simulink model "EvBoltCalib_Lat_v1_comb"  (R2022b)
settings: configuration reference "ConfigSetDesktopFixedStep" (kept outside this file)
PreLoadFcn:
  | VSS_BICYCLE=Simulink.Variant('Dual=0');
  | VSS_DUAL=Simulink.Variant('Dual=1');
  | Dual=1;
undefined symbols (not defined in the file or in its folder): BattChargeLimitMaxPwr, BattChargeLimitSocBpts, BattChargeLimitTbl, BattChrgCapcty, BattDischargeLimitSocBpts, BattDischargeLimitTbl, BattDischargeMaxPwr, BattNumCellsParallel, BattNumCellsSeries, BattOpenVoltCapBpts, BattOpenVoltTbl, BattResistSocBpts, BattResistTbl, BattResistTempBpts, BrakeMaxPrs, BrakeMaxTrq, ChassisDistCg2FrontAxle, ChassisDistCg2RearAxle, ChassisVehMass, DiffRatio, EnvGravCnst, EnvPrs, EnvTemp, ExpRefStructs, FuelSpecificGrav, h, InitStates, MtrEffSpdBpts, MtrEffTbl, MtrEffTrqBpts, MtrPwrMax, MtrTrqMax, SupvsryCtrlRegenBrkCutOffTbl, SupvsryCtrlRegenSpdBpts, TestScnrioCycleNum, VEH
libraries: vehdynlibtire x8, vehdynlibsuspension x7, autolibshared x6, simulink x6, autolibutils x5, VsrLibWheel x4, vehdynlibtirecommon x3, sharedtransform x3, autolibbatterycommon x2, autolibpowerinfoutils x2, autolibsharedcoupling x2, LibPtSupervisoryCtrl x2
(part 1 of 9)
settings Model: DataDictionary=DdPassengerEv.sldd  EnableAccessToBaseWorkspace=off  SimulationMode=accelerator  PauseTimes=45  Creator=9bt  LastModifiedBy=4qz
settings ConfigSetRef: SourceName=ConfigSetDesktopFixedStep

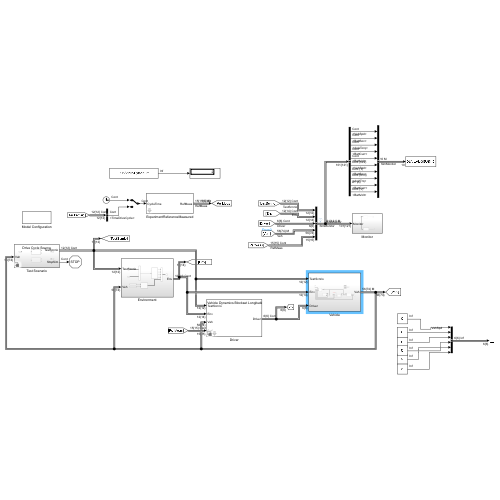
[thumbnail: Simulink's stored preview of the top-level diagram]
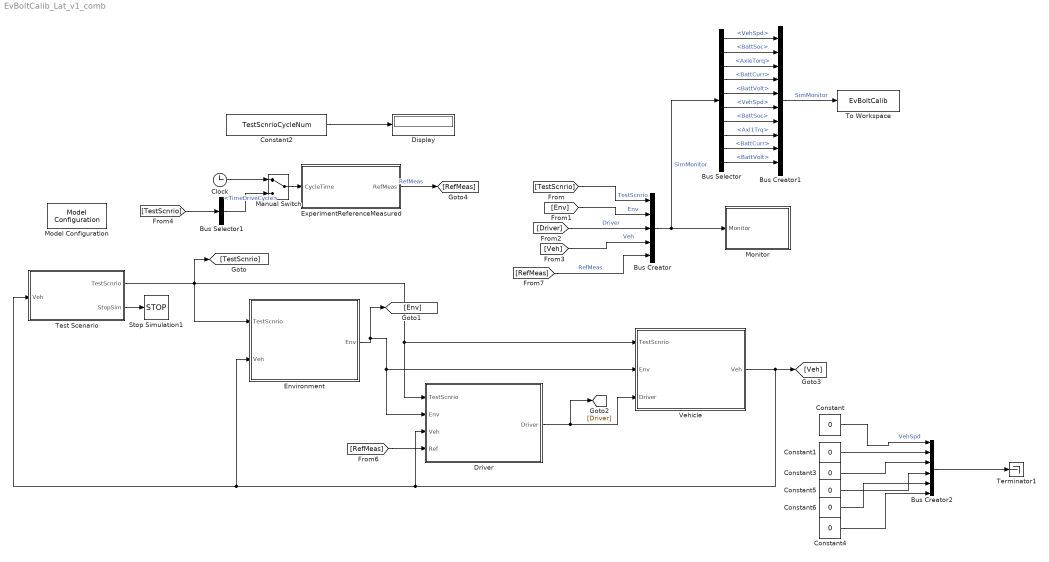
== system EvBoltCalib_Lat_v1_comb ==
  Bus Creator : BusCreator  Inputs=5
  Bus Creator1 : BusCreator  Inputs=10
  Bus Creator2 : BusCreator  Inputs=6
  Bus Selector : BusSelector  OutputSignals=RefMeas.VehSpd,RefMeas.BattSoc,RefMeas.AxleTorq,RefMeas.BattCurr,RefMeas.BattVolt,Veh.Chassis.VehSpd,Veh.Batt.BattSoc,Veh.Diff.Axl1.Axl1Trq,Veh.Batt.BattCurr,Veh.Batt.BattVolt
  Bus Selector1 : BusSelector  OutputSignals=TimeDriveCycle
  Clock : Clock
  Constant{,1,3..6} (6 alike) : Constant  Value=0
  Constant2 : Constant  Value=TestScnrioCycleNum
  Display : Display
  Driver : Subsystem  Variant=on  VariantControlMode=label  LabelModeActiveChoice=VdbLongDriver  mask{DriverSel=Vehicle Dynamics Blockset Longitudinal Driver}
      mask prompts: DriverSel "Select the driver"
      mask init:
      | choice = get_param(gcb,'DriverSel');
      | vssBlk = gcb;
      | oldVariant = get_param(gcb,'LabelModeActiveChoice');
      | switch choice
      |     case 'Predictive Longitudinal Driver'
      |         set_param(vssBlk, 'LabelModeActiveChoice', 'PredDriver');
      |     case 'Open Loop Driver'   
      |         set_param(vssBlk, 'LabelModeActiveChoice', 'OpenLoopDriver');
      |     case 'Direct Command From Reference'   
      |         set_param(vssBlk, 'LabelModeActiveChoice', 'DirectRef');
      |     case 'Vehicle Dynamics Blockset Longitudinal Driver'   
      |         set_param(vssBlk, 'LabelModeActiveChoice', 'VdbLongDriver');
      |     case 'Vehicle Dynamics Blockset Complete Driver'   
      |         set_param(vssBlk, 'LabelModeActiveChoice', 'VdbCompDriver');  
      | end
      mask TypeOptions DriverSel: Predictive Longitudinal Driver | Open Loop Driver | Direct Command From Reference | Vehicle Dynamics Blockset Longitudinal Driver | Vehicle Dynamics Blockset Complete Driver
  Environment : Subsystem
  ExperimentReferenceMeasured : Subsystem  mask{TestScnrioCycleNum=TestScnrioCycleNum, ExpRefStructs=ExpRefStructs}
      mask prompts: TestScnrioCycleNum "Driving Cycle Number"; ExpRefStructs "Experiment Reference Struct from Data Dictionary"
      mask init:
      | obj = ExpRefBlkCtrl(gcb);
      | MaskData = obj.Init;
      mask DialogControl Container3 Prompt: Parameters
  Manual Switch : ManualSwitch
  Model Configuration : VsrLibMdlConfig/Model Configuration  ConfigFileName=getMdlConfigs
  Monitor : Subsystem
  Stop Simulation1 : Stop
  Terminator1 : Terminator
  Test Scenario : Subsystem  Variant=on  VariantControlMode=label  LabelModeActiveChoice=DriveCycleSrc
  To Workspace : ToWorkspace  VariableName=EvBoltCalib  SaveFormat=Structure With Time  SampleTime=-1
  Vehicle : Subsystem
  wires:
  Driver/1(Driver) -> [Driver], Vehicle/3(Driver)
  Environment/1(Env) -> [Env], Driver/2(Env), Vehicle/2(Env)
  [TestScnrio] -> Bus Creator/1  "TestScnrio"
  [Env] -> Bus Creator/2  "Env"
  Test Scenario/2(StopSim) -> Stop Simulation1/1
  [RefMeas] -> Bus Creator/5  "RefMeas"
  Test Scenario/1(TestScnrio) -> [TestScnrio], Driver/1(TestScnrio), Vehicle/1(TestScnrio), Environment/1(TestScnrio)
  [RefMeas] -> Driver/4(Ref)
  ExperimentReferenceMeasured/1(RefMeas) -> [RefMeas]  "RefMeas"
  [TestScnrio] -> Bus Selector1/1
  Manual Switch/1 -> ExperimentReferenceMeasured/1(CycleTime)
  Clock/1 -> Manual Switch/1
  Bus Selector1/1 -> Manual Switch/2  "<TimeDriveCycle>"
  Constant2/1 -> Display/1
  Bus Selector/5 -> Bus Creator1/5  "<BattVolt>"
  Bus Creator1/1 -> To Workspace/1  "SimMonitor"
  Bus Selector/6 -> Bus Creator1/6  "<VehSpd>"
  Bus Selector/10 -> Bus Creator1/10  "<BattVolt>"
  Bus Selector/7 -> Bus Creator1/7  "<BattSoc>"
  Bus Selector/8 -> Bus Creator1/8  "<Axl1Trq>"
  Bus Selector/4 -> Bus Creator1/4  "<BattCurr>"
  Bus Selector/2 -> Bus Creator1/2  "<BattSoc>"
  Bus Selector/3 -> Bus Creator1/3  "<AxleTorq>"
  Bus Selector/1 -> Bus Creator1/1  "<VehSpd>"
  Bus Selector/9 -> Bus Creator1/9  "<BattCurr>"
  Bus Creator/1 -> Monitor/1(Monitor), Bus Selector/1  "SimMonitor"
  [Driver] -> Bus Creator/3  "Driver"
  [Veh] -> Bus Creator/4  "Veh"
  Constant/1 -> Bus Creator2/1  "VehSpd"
  Vehicle/1(Veh) -> Environment/2(Veh), Test Scenario/1(Veh), Driver/3(Veh), [Veh]
  Constant1/1 -> Bus Creator2/2
  Constant3/1 -> Bus Creator2/3
  Constant4/1 -> Bus Creator2/6
  Constant5/1 -> Bus Creator2/4
  Constant6/1 -> Bus Creator2/5
  Bus Creator2/1 -> Terminator1/1

== system EvBoltCalib_Lat_v1_comb/Driver ==
  TestScnrio : Inport
  Env : Inport  Port=2
  Veh : Inport  Port=3
  Ref : Inport  Port=4
  Direct Command From Reference : Subsystem  VariantControl=DirectRef
  Open Loop Driver : Subsystem  VariantControl=OpenLoopDriver
  Predictive Longitudinal Driver : Subsystem  VariantControl=PredDriver
  Vehicle Dynamics Blockset Complete Driver : Subsystem  VariantControl=VdbCompDriver
  "Vehicle Dynamics Blockset Longitudinal Driver " : Subsystem  VariantControl=VdbLongDriver
  Driver : Outport

== system EvBoltCalib_Lat_v1_comb/Environment ==
  TestScnrio : Inport
  Veh : Inport  Port=2
  Friction : Constant  Value=ones(4,1).*1
  Ground Feedback : Subsystem  Variant=on  VariantControlMode=label  LabelModeActiveChoice=0
  Ground Z Level : Constant  Value=zeros(4,1)
  Subsystem : Subsystem
  Subsystem1 : Subsystem
      mask Display: disp('')
  Subsystem2 : Subsystem
      mask Display: disp('')
  Env : Outport
  wires:
  Veh/1 -> Subsystem2/2(Veh)
  Subsystem/3(WindVel) -> Subsystem1/3(WindVel)
  Subsystem/2(EnvTemp) -> Subsystem1/2(EnvTemp)
  Subsystem/4(RoadGrade) -> Subsystem1/4(RoadGrade)
  Subsystem/1(EnvPrs) -> Subsystem1/1(EnvPrs)
  Subsystem1/1(Env) -> Env/1
  TestScnrio/1 -> Subsystem2/1(TestScnrio)
  Subsystem2/1(Grade) -> Subsystem/1(Grade)
  Friction/1 -> Ground Feedback/1(Friction)
  Ground Feedback/1(Ground) -> Subsystem1/5(GroundBus)  "Gnd"
  Ground Z Level/1 -> Ground Feedback/2(Ground Z Level)

== system EvBoltCalib_Lat_v1_comb/ExperimentReferenceMeasured ==
  CycleTime : Inport
  ExpRefLookup : Subsystem
  RefMeas : Outport
  wires:
  CycleTime/1 -> ExpRefLookup/1(CycleTime)
  ExpRefLookup/1(RefMeas) -> RefMeas/1

== system EvBoltCalib_Lat_v1_comb/Monitor ==
  Monitor : Inport
  Calculate Fuel MPG : Subsystem  Commented=on
  Calculate Powertrain Energy : Subsystem
  Terminator : Terminator
  Terminator3 : Terminator
  wires:
  Calculate Fuel MPG/1(FuelEconMPG) -> Terminator/1  "FuelEconMpg"
  Monitor/1 -> Calculate Powertrain Energy/1(Monitor), Calculate Fuel MPG/1(Monitor)
  Calculate Powertrain Energy/1(TransEnrgyOutkWh) -> Terminator3/1  "DiffEnrgyInkWh"

== system EvBoltCalib_Lat_v1_comb/Test Scenario ==
  Veh : Inport
  Drive Cycle Source : Subsystem  VariantControl=DriveCycleSrc
  Open Loop 0-60-0 : Subsystem  VariantControl=OpenLoop0to60to0
  TestScnrio : Outport
  StopSim : Outport  Port=2

== system EvBoltCalib_Lat_v1_comb/Vehicle ==
  TestScnrio : Inport
  Env : Inport  Port=2
  Driver : Inport  Port=3
  Battery : Subsystem
  Bus Creator : BusCreator  Inputs=6
  Bus Selector : BusSelector  OutputSignals=Omega
  Front Wheel Drive : Subsystem  Variant=on  VariantControlMode=label  VariantControl=1  LabelModeActiveChoice=1
  Motor : Subsystem
  "Powertrain Supervisory Controller " : Subsystem  AncestorBlock=LibPtSupervisoryCtrl/Powertrain Supervisory Controller
      settings: LibrarySourceBlock=LibPtSupervisoryCtrl/Powertrain Supervisory Controller
  Terminator : Terminator
  Vehicle Dynamics : Subsystem  Variant=on  VariantControlMode=label  LabelModeActiveChoice=Veh14DOF  mask{VehDynSel=Vehicle 14DOF}
      mask prompts: VehDynSel "Select the driver"
      mask init:
      | choice = get_param(gcb,'VehDynSel');
      | curBlk = gcb;
      | oldVariant = get_param(gcb,'LabelModeActiveChoice');
      | switch choice
      |     case 'Vehicle Longitudinal'
      |         set_param(curBlk, 'LabelModeActiveChoice', 'VehLong');
      | %     case 'Vehicle 3DOF'   
      | %         set_param(curBlk, 'LabelModeActiveChoice', 'Veh3DOF');
      |     case 'Vehicle 7DOF'   
      |         set_param(curBlk, 'LabelModeActiveChoice', 'Veh7DOF');
      |     case 'Vehicle 14DOF'   
      |         set_param(curBlk, 'LabelModeActiveChoice', 'Veh14DOF');
      | end
      mask TypeOptions VehDynSel: Vehicle Longitudinal | Vehicle 7DOF | Vehicle 14DOF
  Veh : Outport
  wires:
  "Powertrain Supervisory Controller "/1(SupvsryCtrl) -> Vehicle Dynamics/2(SupvsryCtrl), Motor/1(SupvsryCtrl), [SupvsryCtrl]
  Driver/1 -> "Powertrain Supervisory Controller "/1(Driver)
  Bus Creator/1 -> Veh/1  "Veh"
  TestScnrio/1 -> Terminator/1
  [SupvsryCtrl] -> Bus Creator/1  "SupvsryCtrl"
  [Batt] -> Bus Creator/2  "Batt"
  [Mtr] -> Bus Creator/3  "Mtr"
  [Whl] -> Bus Creator/5  "Whl"
  [Chassis] -> Bus Creator/6  "Chassis"
  Battery/1(Batt) -> "Powertrain Supervisory Controller "/4(Batt), [Batt]
  Motor/1(Mtr) -> "Powertrain Supervisory Controller "/3(Mtr), [Mtr]
  Env/1 -> Vehicle Dynamics/1(Env)
  Vehicle Dynamics/2(Chassis) -> "Powertrain Supervisory Controller "/2(Chassis), [Chassis]
  Vehicle Dynamics/1(Whl) -> [Whl]
  [Whl] -> Bus Selector/1
  [Diff] -> Bus Creator/4  "Diff"
  Bus Selector/1 -> Front Wheel Drive/2(Omega)  "<Omega>"
  Front Wheel Drive/1(Diff) -> [Diff]
  Front Wheel Drive/2(AxlTrq) -> Vehicle Dynamics/3(AxlTrq)
  Front Wheel Drive/3(PropShaftSpd) -> Motor/2(MtrSpd)
  Motor/2(MtrTrq) -> Front Wheel Drive/1(DrvShfTrq)
  connections:
  Battery/RConn1 -- Motor/LConn1

== system EvBoltCalib_Lat_v1_comb/Driver/Direct Command From Reference ==
  TestScnrio : Inport
  Env : Inport  Port=2
  Veh : Inport  Port=3
  Ref : Inport  Port=4
  Bus Selector1 : BusSelector  OutputSignals=AccelPedalCmd,BrakePedalCmd
  Bus Selector2 : BusSelector  OutputSignals=LatRef.Steering
  Constant : Constant
  Constant1 : Constant
  Constant2 : Constant  Value=0
  Subsystem1 : Subsystem
      mask Display: disp('')
  Subsystem2 : Subsystem
      mask Display: disp('')
  Driver : Outport
  wires:
  Constant1/1 -> Subsystem1/3(GearCmd)
  Subsystem1/1(TransPlant) -> Driver/1
  Bus Selector1/2 -> Subsystem1/2(DecelCmd)  "<BrakePedalCmd>"
  Bus Selector1/1 -> Subsystem1/1(AccelCmd)  "<AccelPedalCmd>"
  Constant2/1 -> Subsystem1/4(CltchCmd)
  Ref/1 -> Bus Selector1/1
  Constant/1 -> Subsystem1/5(IgSw)
  Env/1 -> Subsystem2/1(Env)
  Veh/1 -> Subsystem2/2(Veh)
  TestScnrio/1 -> Bus Selector2/1
  Bus Selector2/1 -> Subsystem1/6(SteeringCmd)  "<Steering>"

== system EvBoltCalib_Lat_v1_comb/Driver/Open Loop Driver ==
  TestScnrio : Inport
  Env : Inport  Port=2
  Veh : Inport  Port=3
  Ref : Inport  Port=4
  Constant : Constant  Value=0
  Longitudinal Driver : Subsystem
  Subsystem1 : Subsystem
      mask Display: disp('')
  Subsystem2 : Subsystem
      mask Display: disp('')
  Terminator : Terminator
  Driver : Outport
  wires:
  Subsystem2/2(DecelCmd) -> Longitudinal Driver/2(DecelCmdIn)
  Subsystem2/1(AccelCmd) -> Longitudinal Driver/1(AccelCmdIn)
  Veh/1 -> Subsystem2/3(Veh)
  Env/1 -> Subsystem2/2(Env)
  TestScnrio/1 -> Subsystem2/1(TestScnrio)
  Subsystem1/1(TransPlant) -> Driver/1
  Longitudinal Driver/5(IgSw) -> Subsystem1/5(IgSw)
  Longitudinal Driver/1(AccelCmd) -> Subsystem1/1(AccelCmd)
  Longitudinal Driver/4(CltchCmd) -> Subsystem1/4(CltchCmd)
  Longitudinal Driver/2(DecelCmd) -> Subsystem1/2(DecelCmd)
  Longitudinal Driver/3(GearCmd) -> Subsystem1/3(GearCmd)
  Ref/1 -> Terminator/1
  Constant/1 -> Subsystem1/6(SteeringCmd)

== system EvBoltCalib_Lat_v1_comb/Driver/Predictive Longitudinal Driver ==
  TestScnrio : Inport
  Env : Inport  Port=2
  Veh : Inport  Port=3
  Ref : Inport  Port=4
  Constant : Constant  Value=0
  Longitudinal Driver : Subsystem
  Subsystem1 : Subsystem
      mask Display: disp('')
  Subsystem2 : Subsystem
      mask Display: disp('')
  Terminator : Terminator
  Driver : Outport
  wires:
  Longitudinal Driver/3(GearCmd) -> Subsystem1/3(GearCmd)
  Longitudinal Driver/2(DecelCmd) -> Subsystem1/2(DecelCmd)
  Longitudinal Driver/4(CltchCmd) -> Subsystem1/4(CltchCmd)
  Longitudinal Driver/1(AccelCmd) -> Subsystem1/1(AccelCmd)
  Longitudinal Driver/5(IgSw) -> Subsystem1/5(IgSw)
  Subsystem1/1(TransPlant) -> Driver/1
  TestScnrio/1 -> Subsystem2/1(TestScnrio)
  Env/1 -> Subsystem2/2(Env)
  Veh/1 -> Subsystem2/3(Veh)
  Subsystem2/1(VehRefSpd) -> Longitudinal Driver/1(VehRefSpd)
  Subsystem2/2(VehRefSpdLookAhead) -> Longitudinal Driver/2(VehRefSpdLookAhead)
  Subsystem2/3(VehDistLookAhead) -> Longitudinal Driver/3(VehDistLookAhead)
  Subsystem2/4(TimeLookAhead) -> Longitudinal Driver/4(TimeLookAhead)
  Subsystem2/5(VehSpd) -> Longitudinal Driver/5(VehSpd)
  Subsystem2/6(VehDist) -> Longitudinal Driver/6(VehDist)
  Subsystem2/7(RoadGrade) -> Longitudinal Driver/7(RoadGrade)
  Subsystem2/8(GradeLookAhead) -> Longitudinal Driver/8(GradeLookAhead)
  Ref/1 -> Terminator/1
  Constant/1 -> Subsystem1/6(SteeringCmd)

== system EvBoltCalib_Lat_v1_comb/Driver/Vehicle Dynamics Blockset Complete Driver ==
  TestScnrio : Inport
  Env : Inport  Port=2
  Veh : Inport  Port=3
  Ref : Inport  Port=4
  Complete Driver : Subsystem
  Subsystem3 : Subsystem
      mask Display: disp('')
  Terminator : Terminator
  Driver : Outport
  wires:
  TestScnrio/1 -> Complete Driver/1(TestScnrio)
  Env/1 -> Complete Driver/2(Env)
  Veh/1 -> Complete Driver/3(Veh)
  Ref/1 -> Terminator/1
  Complete Driver/1(AccelCmd) -> Subsystem3/1(AccelCmd)
  Subsystem3/1(TransPlant) -> Driver/1
  Complete Driver/4(CltchCmd) -> Subsystem3/4(CltchCmd)
  Complete Driver/2(DecelCmd) -> Subsystem3/2(DecelCmd)
  Complete Driver/3(GearCmd) -> Subsystem3/3(GearCmd)
  Complete Driver/5(IgSw) -> Subsystem3/5(IgSw)
  Complete Driver/6(SteerCmd) -> Subsystem3/6(SteeringCmd)

== system EvBoltCalib_Lat_v1_comb/Driver/Vehicle Dynamics Blockset Longitudinal Driver  ==
  TestScnrio : Inport
  Env : Inport  Port=2
  Veh : Inport  Port=3
  Ref : Inport  Port=4
  Constant : Constant  Value=0
  Longitudinal Driver : Subsystem
  Subsystem1 : Subsystem
      mask Display: disp('')
  Subsystem2 : Subsystem
      mask Display: disp('')
  Terminator : Terminator
  Driver : Outport
  wires:
  Longitudinal Driver/3(GearCmd) -> Subsystem1/3(GearCmd)
  Longitudinal Driver/2(DecelCmd) -> Subsystem1/2(DecelCmd)
  Longitudinal Driver/4(CltchCmd) -> Subsystem1/4(CltchCmd)
  Longitudinal Driver/1(AccelCmd) -> Subsystem1/1(AccelCmd)
  Longitudinal Driver/5(IgSw) -> Subsystem1/5(IgSw)
  Subsystem1/1(TransPlant) -> Driver/1
  TestScnrio/1 -> Subsystem2/1(TestScnrio)
  Env/1 -> Subsystem2/2(Env)
  Veh/1 -> Subsystem2/3(Veh)
  Subsystem2/1(VehRefSpd) -> Longitudinal Driver/1(VehRefSpd)
  Subsystem2/2(VehRefSpdLookAhead) -> Longitudinal Driver/2(VehRefSpdLookAhead)
  Subsystem2/3(VehDistLookAhead) -> Longitudinal Driver/3(VehDistLookAhead)
  Subsystem2/4(TimeLookAhead) -> Longitudinal Driver/4(TimeLookAhead)
  Subsystem2/5(VehSpd) -> Longitudinal Driver/5(VehSpd)
  Subsystem2/6(VehDist) -> Longitudinal Driver/6(VehDist)
  Subsystem2/7(RoadGrade) -> Longitudinal Driver/7(RoadGrade)
  Subsystem2/8(GradeLookAhead) -> Longitudinal Driver/8(GradeLookAhead)
  Ref/1 -> Terminator/1
  Constant/1 -> Subsystem1/6(SteeringCmd)

== system EvBoltCalib_Lat_v1_comb/Environment/Ground Feedback ==
  note: 1) Add Subsystem or Model blocks as valid variant choices.
      | 2) You cannot connect blocks at this level. At simulation, connectivity is automatically
      | determined, based on the active variant and port name matching.
  Friction : Inport
  Ground Z Level : Inport  Port=2
  3D Engine : Subsystem  VariantControl=1
  Constant : Subsystem  VariantControl=0
  Ground : Outport  VectorParamsAs1DForOutWhenUnconnected=off

== system EvBoltCalib_Lat_v1_comb/Environment/Subsystem ==
  Grade : Inport
  Constant : Constant  Value=EnvPrs
  Constant1 : Constant  Value=EnvTemp
  Constant2 : Constant  Value=0
  Constant3 : Constant  Value=0
  Constant4 : Constant  Value=0
  Signal Specification : SignalSpecification  Unit=Pa
  Signal Specification1 : SignalSpecification  Unit=K
  Signal Specification2 : SignalSpecification  Unit=rad
  Signal Specification3 : SignalSpecification  Unit=m/s
  Signal Specification4 : SignalSpecification  Unit=m/s
  Signal Specification5 : SignalSpecification  Unit=m/s
  Vector Concatenate : Concatenate  NumInputs=3
  EnvPrs : Outport
  EnvTemp : Outport  Port=2
  WindVel : Outport  Port=3
  RoadGrade : Outport  Port=4
  wires:
  Constant/1 -> Signal Specification/1
  Constant2/1 -> Signal Specification3/1
  Constant1/1 -> Signal Specification1/1
  Grade/1 -> Signal Specification2/1
  Signal Specification/1 -> EnvPrs/1
  Signal Specification1/1 -> EnvTemp/1
  Signal Specification2/1 -> RoadGrade/1
  Vector Concatenate/1 -> WindVel/1
  Signal Specification3/1 -> Vector Concatenate/1  "WindX"
  Constant3/1 -> Signal Specification4/1
  Constant4/1 -> Signal Specification5/1
  Signal Specification4/1 -> Vector Concatenate/2  "WindY"
  Signal Specification5/1 -> Vector Concatenate/3  "WindZ"

== system EvBoltCalib_Lat_v1_comb/Environment/Subsystem1 ==
  EnvPrs : Inport
  EnvTemp : Inport  Port=2
  WindVel : Inport  Port=3
  RoadGrade : Inport  Port=4
  GroundBus : Inport  Port=5
  Bus Creator : BusCreator  Inputs=5
  Env : Outport
  wires:
  EnvPrs/1 -> Bus Creator/1  "EnvPrs"
  EnvTemp/1 -> Bus Creator/2  "EnvTemp"
  Bus Creator/1 -> Env/1  "Env"
  WindVel/1 -> Bus Creator/3  "WindVel"
  RoadGrade/1 -> Bus Creator/4  "RoadGrade"
  GroundBus/1 -> Bus Creator/5  "GndBus"

== system EvBoltCalib_Lat_v1_comb/Environment/Subsystem2 ==
  TestScnrio : Inport
  Veh : Inport  Port=2
  Bus Selector : BusSelector  OutputSignals=Grade
  Terminator1 : Terminator
  Grade : Outport
  wires:
  TestScnrio/1 -> Bus Selector/1
  Bus Selector/1 -> Grade/1  "<Grade>"
  Veh/1 -> Terminator1/1

== system EvBoltCalib_Lat_v1_comb/ExperimentReferenceMeasured/ExpRefLookup ==
  CycleTime : Inport
  APP (0,1) : Lookup_n-D  NumberOfTableDimensions=1  BreakpointsForDimension1=MaskData.time  Table=MaskData.accelPedalCmd  InternalRulePriority=Speed  RndMeth=Simplest
  APP_DBW (0,1) : Lookup_n-D  NumberOfTableDimensions=1  BreakpointsForDimension1=MaskData.time  Table=MaskData.accelPedalDBW  InternalRulePriority=Speed  RndMeth=Simplest
  Axle_Torque : Lookup_n-D  NumberOfTableDimensions=1  BreakpointsForDimension1=MaskData.time  Table=MaskData.axleTorq  InternalRulePriority=Speed  RndMeth=Simplest
  BPP (0,1) : Lookup_n-D  NumberOfTableDimensions=1  BreakpointsForDimension1=MaskData.time  Table=MaskData.brakePedalCmd  InternalRulePriority=Speed  RndMeth=Simplest
  BPP_DBW (0,1) : Lookup_n-D  NumberOfTableDimensions=1  BreakpointsForDimension1=MaskData.time  Table=MaskData.brakePedalDBW  InternalRulePriority=Speed  RndMeth=Simplest
  Battery SOC (0,1) : Lookup_n-D  NumberOfTableDimensions=1  BreakpointsForDimension1=MaskData.time  Table=MaskData.battSoc  InternalRulePriority=Speed  RndMeth=Simplest
  Battery Voltage : Lookup_n-D  NumberOfTableDimensions=1  BreakpointsForDimension1=MaskData.time  Table=MaskData.battVolt  InternalRulePriority=Speed  RndMeth=Simplest
  Battery_Current : Lookup_n-D  NumberOfTableDimensions=1  BreakpointsForDimension1=MaskData.time  Table=MaskData.battCurr  InternalRulePriority=Speed  RndMeth=Simplest
  Brake Torque : Lookup_n-D  NumberOfTableDimensions=1  BreakpointsForDimension1=MaskData.time  Table=MaskData.brakeTorq  InternalRulePriority=Speed  RndMeth=Simplest
  Bus Creator : BusCreator  Inputs=15
  Grade (rad) : Lookup_n-D  NumberOfTableDimensions=1  BreakpointsForDimension1=MaskData.time  Table=MaskData.grade  InternalRulePriority=Speed  RndMeth=Simplest
  Velocity (m/s) : Lookup_n-D  NumberOfTableDimensions=1  BreakpointsForDimension1=MaskData.time  Table=MaskData.vehSpd  InternalRulePriority=Speed  RndMeth=Simplest
  refSpare3 : Lookup_n-D  NumberOfTableDimensions=1  BreakpointsForDimension1=MaskData.time  Table=MaskData.spare3  InternalRulePriority=Speed  RndMeth=Simplest
  refSpare4 : Lookup_n-D  NumberOfTableDimensions=1  BreakpointsForDimension1=MaskData.time  Table=MaskData.spare4  InternalRulePriority=Speed  RndMeth=Simplest
  refSpare5 : Lookup_n-D  NumberOfTableDimensions=1  BreakpointsForDimension1=MaskData.time  Table=MaskData.spare5  InternalRulePriority=Speed  RndMeth=Simplest
  refSpare6 : Lookup_n-D  NumberOfTableDimensions=1  BreakpointsForDimension1=MaskData.time  Table=MaskData.spare6  InternalRulePriority=Speed  RndMeth=Simplest
  RefMeas : Outport
  wires:
  CycleTime/1 -> refSpare4/1, refSpare5/1, refSpare6/1, refSpare3/1, Brake Torque/1, Grade (rad)/1, Axle_Torque/1, Battery_Current/1, Battery Voltage/1, Battery SOC (0,1)/1, Velocity (m/s)/1, BPP_DBW (0,1)/1, APP_DBW (0,1)/1, BPP (0,1)/1, APP (0,1)/1
  refSpare3/1 -> Bus Creator/12  "Spare3"
  Velocity (m/s)/1 -> Bus Creator/5  "VehSpd"
  Battery Voltage/1 -> Bus Creator/7  "BattVolt"
  Axle_Torque/1 -> Bus Creator/9  "AxleTorq"
  refSpare6/1 -> Bus Creator/15  "Spare6"
  APP (0,1)/1 -> Bus Creator/1  "AccelPedalCmd"
  Grade (rad)/1 -> Bus Creator/10  "Grade"
  Battery SOC (0,1)/1 -> Bus Creator/6  "BattSoc"
  Brake Torque/1 -> Bus Creator/11  "BrakeTorq"
  refSpare5/1 -> Bus Creator/14  "Spare5"
  BPP_DBW (0,1)/1 -> Bus Creator/4  "BrakePredalDBW"
  Battery_Current/1 -> Bus Creator/8  "BattCurr"
  refSpare4/1 -> Bus Creator/13  "Spare4"
  APP_DBW (0,1)/1 -> Bus Creator/3  "AccelPedalDBW"
  BPP (0,1)/1 -> Bus Creator/2  "BrakePedalCmd"
  Bus Creator/1 -> RefMeas/1

== system EvBoltCalib_Lat_v1_comb/Monitor/Calculate Fuel MPG ==
  Monitor : Inport
  Bus Selector : BusSelector  OutputSignals=Veh.Chassis.VehDist,Veh.Batt.EngPlant.FuellMassFlw
  Constant : Constant  Value=FuelSpecificGrav
  Density of Water : Gain  Gain=997
  Divide : Product  Inputs=*/
  Divide1 : Product  Inputs=*/
  Integrator : Integrator
  Saturation : Saturate  UpperLimit=inf  LowerLimit=1e-7
  Signal Specification : SignalSpecification  Unit=mi
  Signal Specification1 : SignalSpecification  Unit=m^3
  Signal Specification2 : SignalSpecification  Unit=gal
  Unit Conversion : UnitConversion
  Unit Conversion1 : UnitConversion
  FuelEconMPG : Outport
  wires:
  Divide1/1 -> FuelEconMPG/1  "FuelEconMPG"
  Divide/1 -> Signal Specification1/1
  Unit Conversion1/1 -> Signal Specification2/1
  Signal Specification2/1 -> Saturation/1
  Unit Conversion/1 -> Signal Specification/1
  Bus Selector/1 -> Unit Conversion/1  "<VehDist>"
  Bus Selector/2 -> Integrator/1  "<FuellMassFlw>"
  Integrator/1 -> Divide/1  "FuelMass"
  Density of Water/1 -> Divide/2
  Saturation/1 -> Divide1/2  "FuelVolume"
  Constant/1 -> Density of Water/1
  Signal Specification1/1 -> Unit Conversion1/1
  Monitor/1 -> Bus Selector/1
  Signal Specification/1 -> Divide1/1  "VehDistMiles"

== system EvBoltCalib_Lat_v1_comb/Monitor/Calculate Powertrain Energy ==
  Monitor : Inport
  Bus Selector2 : BusSelector  OutputSignals=Veh.Diff.PwrInfo.PwrTrnsfrd.PwrTrnsfrd.PwrDriveshft
  Integrator : Integrator
  Signal Specification : SignalSpecification  Unit=J
  Signal Specification1 : SignalSpecification  Unit=kW*h
  Unit Conversion : UnitConversion
  TransEnrgyOutkWh : Outport
  wires:
  Unit Conversion/1 -> Signal Specification1/1
  Integrator/1 -> Signal Specification/1  "EnrgyTrans"
  Signal Specification/1 -> Unit Conversion/1
  Signal Specification1/1 -> TransEnrgyOutkWh/1
  Monitor/1 -> Bus Selector2/1
  Bus Selector2/1 -> Integrator/1  "<PwrDriveshft>"

== system EvBoltCalib_Lat_v1_comb/Test Scenario/Drive Cycle Source ==
  Veh : Inport
  Bus Creator : BusCreator  Inputs=11
  Bus Selector : BusSelector  OutputSignals=Chassis.VehSpd
  Bus Selector1 : BusSelector  OutputSignals=VehRefSpdLookAhead,GradeLookAhead,TimeLookAhead,DriveCycleDist,VehDist,VehDistLookAhead,TimeDriveCycle
  Constant : Constant
  Constant1 : Constant
  Constant2 : Constant  Value=TestScnrioCycleNum
  LatCoGDispRef : Constant  Value=0
  SteeringRef : Constant  Value=0
  Subsystem1 : Subsystem
      mask Display: disp('')
  VSR Drive Cycle Source : VsrLibDriveCycleSrc/VSR Drive Cycle Source  DistCompensationCheckbox=off  DriveCycleStructArray=TestScnrioDriveCycleStructs  TimeLookAhead=0
  TestScnrio : Outport
  StopSim : Outport  Port=2
  wires:
  VSR Drive Cycle Source/2 -> Bus Creator/1  "VehRefSpd"
  Bus Creator/1 -> TestScnrio/1  "TestScenario"
  Veh/1 -> Bus Selector/1
  VSR Drive Cycle Source/4 -> StopSim/1, Bus Creator/9  "CycleCompleted"
  VSR Drive Cycle Source/1 -> Bus Selector1/1
  Bus Selector/1 -> VSR Drive Cycle Source/1  "<VehSpd>"
  Constant/1 -> VSR Drive Cycle Source/2
  Constant1/1 -> VSR Drive Cycle Source/3
  Constant2/1 -> VSR Drive Cycle Source/4
  VSR Drive Cycle Source/3 -> Bus Creator/3  "Grade"
  Bus Selector1/1 -> Bus Creator/2  "<VehRefSpdLookAhead>"
  Bus Selector1/2 -> Bus Creator/4  "<GradeLookAhead>"
  Bus Selector1/3 -> Bus Creator/5  "<TimeLookAhead>"
  Bus Selector1/4 -> Bus Creator/6  "<DriveCycleDist>"
  Bus Selector1/6 -> Bus Creator/8  "<VehDistLookAhead>"
  Bus Selector1/5 -> Bus Creator/7  "<VehDist>"
  Bus Selector1/7 -> Bus Creator/10  "<TimeDriveCycle>"
  LatCoGDispRef/1 -> Subsystem1/1(LatCoGDispRef)
  SteeringRef/1 -> Subsystem1/2(SteeringRef)
  Subsystem1/1(LatRef) -> Bus Creator/11  "LatRef"

== system EvBoltCalib_Lat_v1_comb/Test Scenario/Open Loop 0-60-0 ==
  Veh : Inport
  Bus Creator : BusCreator  Inputs=3
  Bus Selector : BusSelector  OutputSignals=Chassis.VehSpd
  Chart : Stateflow chart  TreatAsAtomicUnit=on
  Constant : Constant  Value=0
  Signal Specification : SignalSpecification  Unit=mph
  Unit Conversion : UnitConversion
  TestScnrio : Outport
  StopSim : Outport  Port=2
  wires:
  Bus Creator/1 -> TestScnrio/1  "TestScenario"
  Chart/1(AccelCmd) -> Bus Creator/1  "AccelCmd"
  Chart/2(DecelCmd) -> Bus Creator/2  "DecelCmd"
  Veh/1 -> Bus Selector/1
  Bus Selector/1 -> Unit Conversion/1  "<VehSpd>"
  Unit Conversion/1 -> Signal Specification/1
  Signal Specification/1 -> Chart/1(VehSpdMph)  "VehSpdMph"
  Chart/3(StopSim) -> StopSim/1
  Constant/1 -> Bus Creator/3  "Grade"

== system EvBoltCalib_Lat_v1_comb/Vehicle/Battery ==
  Battery : Subsystem
  Subsystem1 : Subsystem
      mask Display: disp('')
  BattOut : PMIOPort  Side=Right
  Batt : Outport
  wires:
  Battery/1(BattSoc) -> Subsystem1/1(BattSoc)
  Battery/2(BattCurr) -> Subsystem1/2(BattCurr)
  Battery/3(BattVolt) -> Subsystem1/3(BattVolt)
  Subsystem1/1(Batt) -> Batt/1
  connections:
  BattOut/RConn1 -- Battery/RConn1

== system EvBoltCalib_Lat_v1_comb/Vehicle/Front Wheel Drive ==
  DrvShfTrq : Inport
  Omega : Inport  Port=2
  Ideal Diff : Subsystem  VariantControl=0
  Real Diff : Subsystem  VariantControl=1
  Diff : Outport  VectorParamsAs1DForOutWhenUnconnected=off
  AxlTrq : Outport  Port=2  VectorParamsAs1DForOutWhenUnconnected=off
  PropShaftSpd : Outport  Port=3  VectorParamsAs1DForOutWhenUnconnected=off

== system EvBoltCalib_Lat_v1_comb/Vehicle/Motor ==
  SupvsryCtrl : Inport
  MtrSpd : Inport  Port=2
  Bus Creator1 : BusCreator  Inputs=1
  Bus Creator2 : BusCreator  Inputs=4
  Bus Selector1 : BusSelector  OutputSignals=Volt
  Bus Selector2 : BusSelector  OutputSignals=MtrTrqCmd
  Bus Selector3 : BusSelector  OutputSignals=PwrInfo.PwrTrnsfrd.PwrMtr,PwrInfo.PwrTrnsfrd.PwrBus
  Mapped Motor : autolibmappedmotor/Mapped Motor  port_config=Speed  param_by=Maximum torque and power  w_t=[ 0 375 750 800 ]  T_t=[0.09 0.08 0.07 0]  torque_max=MtrTrqMax  power_max=MtrPwrMax  Tc=MtrTrqTimeCnst  param_loss=Tabulated efficiency data  eff=100  w_eff=375  T_eff=0.08  Piron=0  Pbase=0  w_eff_bp=MtrEffSpdBpts.*pi/30  T_eff_bp=MtrEffTrqBpts  Temp_eff_bp=[233.15 293.15 373.15]  losses_table=[1 2;3 4]  losses_table_3d=cat(3,[1.49 1.67 2.21 3.10; 0.42 0.69 1.14 2.03; 0.06 0.24 0.78 1.68; 0.42 0.69 1.14 2.03; 1.49 1.67 2.21 3.10],[1.49 1.67 2.21 3.10; 0.42 0.69 1.14 2.03; 0.06 0.24 0.78 1.68; 0.42 0.69 1.14 2.03; 1.49 1.67 2.21 3.10],[1.49 1.67 2.21 3.10; 0.42 0.69 1.14 2.03; 0.06 0.24 0.78 1.68; 0.42 0.69 1.14 2.03; 1.49 1.67 2.21 3.10])  efficiency_table=MtrEffTbl*0.94  efficiency_table_3d=cat(3,[95 95 95 95; 95 95 95 95; 95 95 95 95; 95 95 95 95; 95 95 95 95],[95 95 95 95; 95 95 95 95; 95 95 95 95; 95 95 95 95; 95 95 95 95],[95 95 95 95; 95 95 95 95; 95 95 95 95; 95 95 95 95; 95 95 95 95])  J=5e-6  b=1e-5  omega_o=0  T_t_extended=[0 0.07 0.08 0.09 0.08 0.07 0]  w_t_extended=[-800 -750 -375 0 375 750 800]  KLossIron=0  KLossCopper=0  x_w_eff_vec=[-1047.1975511966 -942.477796076938 -837.758040957278 -733.038285837618 -628.318530717959 -523.598775598299 -418.879020478639 -314.159265358979 -285.714285713875 -209.43951023932 -104.71975511966 0 104.71975511966 209.43951023932 285.714285713875 314.159265358979 418.879020478639 523.598775598299 628.318530717959 733.038285837618 837.758040957278 942.477796076938 1047.1975511966]  x_T_eff_vec=[-360 -334.285714285714 -308.571428571429 -282.857142857143 -257.142857142857 -231.428571428571 -205.714285714286 -180 -154.285714285714 -128.571428571429 -102.857142857143 -77.1428571428572 -51.4285714285714 -25.7142857142857 0 25.7142857142857 51.4285714285714 77.1428571428572 102.857142857143 128.571428571429 154.285714285714 180 205.714285714286 231.428571428571 257.142857142857 282.857142857143 308.571428571429 334.285714285714 360]  x_tmp_eff_vec=[-0.09 -0.06 -0.03 0 0.03 0.06 0.09]  x_losses_mat=[54250.1517943165 50375.1409518653 46500.1301094142 42625.119266963 38750.1084245118 34875.0975820605 31000.0867396095 27125.0758971582 23250.065054707 19375.054212256 15500.0433698047 12629.4764797412 9803.55154311708 6774.11181875432 0 5412.5153431847 8293.80460547705 10921.9712596802 13550.1379138833 16937.6723923542 20325.2068708249 23712.7413492957 27100.2758277666 30487.8103062373 33875.3447847082 37262.879263179 40650.4137416499 44037.9482201206 47425.4826985915;44696.230836134 41503.6429192672 38311.0550024006 35118.4670855338 31925.8791686671 28733.2912518003 25540.7033349337 22348.115418067 19155.5275012002 15962.9395843336 12770.3516674669 9577.76375060014 6975.01951641212 6096.70063687888 0 4871.26380886623 6097.56206124747 8462.91205003029 11283.8827333737 14104.8534167172 16925.8241000605 19746.794783404 22567.7654667475 25388.7361500908 28209.7068334343 31030.6775167777 33851.6482001212 36672.6188834645 39493.589566808;36137.1105685043 33555.8883850397 30974.6662015752 28393.4440181105 25812.2218346459 23230.9996511813 20649.7774677168 18068.5552842522 15487.3331007875 12906.110917323 10324.8887338584 8513.56777831124 6200.01734792188 5419.28945500345 0 4330.01227454776 5420.05516555331 7522.58848891581 9220.12563933554 11525.1570491694 13830.1884590033 16135.2198688372 18440.2512786711 20745.2826885049 23050.3140983388 25355.3455081727 27660.3769180066 29965.4083278404 32270.4397376744;31619.9717474413 29361.4023369097 27102.8329263783 24844.2635158467 22585.6941053152 20327.1246947836 18068.5552842522 15809.9858737206 13551.4164631891 11292.8470526576 9034.27764212609 7449.37180602233 5425.01517943165 4741.87827312802 0 3788.76074022929 4742.54826985915 6582.26492780134 8067.6099344186 10084.5124180233 12101.4149016279 14118.3173852325 16135.2198688372 18152.1223524418 20169.0248360465 22185.9273196511 24202.8298032558 26219.7322868604 28236.6347704651;27102.8329263782 25166.9162887798 23230.9996511814 21295.0830135829 19359.1663759844 17423.249738386 15487.3331007876 13551.4164631891 11615.4998255906 9679.58318799226 8513.56777831124 6385.17583373343 4650.01301094141 4064.46709125259 0 3247.50920591082 4065.04137416498 5641.94136668686 7522.58848891582 8643.86778687709 10372.6413442524 12101.4149016279 13830.1884590033 15558.9620163787 17287.7355737541 19016.5091311295 20745.282688505 22474.0562458803 24202.8298032558;22585.6941053152 20972.4302406498 19359.1663759845 17745.9025113191 16132.6386466537 14519.3747819883 12906.110917323 11292.8470526576 9679.58318799221 8066.31932332688 7094.63981525937 5320.97986144452 3875.01084245118 3387.05590937716 0 2706.25767159235 3387.53447847082 4701.61780557238 6268.82374076318 7203.22315573091 8643.86778687704 10084.5124180232 11525.1570491694 12965.8016803156 14406.4463114618 15847.0909426079 17287.7355737541 18728.3802049003 20169.0248360465;19864.9914827262 18446.0635196743 17027.1355566225 15608.2075935706 14189.2796305187 12770.3516674668 11351.423704415 9932.4957413631 8513.56777831121 7094.63981525938 5675.71185220749 4256.78388915562 3100.00867396094 2709.64472750173 0 2165.00613727388 2710.02758277665 3761.29424445791 5015.05899261055 6268.82374076319 7522.58848891579 8776.35323706844 10030.1179852211 11283.8827333737 12537.6474815263 13791.412229679 15045.1769778316 16298.9417259842 17552.7064741369;20587.4582405459 19116.9255090783 17646.3927776108 16175.8600461432 12629.4764797412 11366.528831767 10103.581183793 8137.52276914747 6975.01951641211 5812.51626367679 4650.01301094142 3788.84294392236 2525.89529594824 2032.23354562629 0 1623.75460295541 2184.39425193603 3276.59137790406 4065.04137416499 5081.30171770625 6097.56206124746 7113.82240478872 8737.57700774416 9829.77413371214 10921.9712596802 13684.7775990372 14928.8482898587 16172.9189806802 17416.9896715018;18723.4042552922 17386.0182370571 16048.6322188219 14711.2462005868 11485.9634880614 10337.3671392553 9188.77079044916 8040.174441643 6891.57809283685 5742.98174403074 4594.38539522458 ...(+6536 chars)]  x_losses_mat_3d=[37.8947368421052 25.2631578947368 12.6315789473684 0 12 24 36;18.9473684210526 12.6315789473684 6.3157894736842 0 5.99999999999999 12 18;0 0 0 0 0 0 0;18 12 5.99999999999999 0 6.3157894736842 12.6315789473684 18.9473684210526;36 24 12 0 12.6315789473684 25.2631578947368 37.8947368421052]  CalLossMapData={}  CalLossWithTempMapData={}  aMode=aMode  RefBlkName='autolibmappedmotor/Mapped Motor'
  Memory : Memory
  Mux{,1..3} (4 alike) : Mux  Inputs=1
  Two-Way Connection1 : TwoWayConnection
  Batt : PMIOPort  Side=Left
  Mtr : Outport
  MtrTrq : Outport  Port=2
  wires:
  Mapped Motor/3 -> Mux/1, MtrTrq/1  "Trq"
  Mapped Motor/2 -> Memory/1  "Curr"
  Bus Creator1/1 -> Two-Way Connection1/1
  Mapped Motor/1 -> Bus Selector3/1
  SupvsryCtrl/1 -> Bus Selector2/1
  Two-Way Connection1/1 -> Bus Selector1/1
  Bus Selector1/1 -> Mapped Motor/1  "<Volt>"
  Bus Selector2/1 -> Mapped Motor/3  "<MtrTrqCmd>"
  Mux/1 -> Bus Creator2/2  "MtrTrq"
  Bus Creator2/1 -> Mtr/1
  Mux2/1 -> Bus Creator2/3  "MtrMechPwr"
  Bus Selector3/1 -> Mux2/1  "<PwrMtr>"
  Mux1/1 -> Bus Creator2/1  "MtrSpd"
  Bus Selector3/2 -> Mux3/1  "<PwrBus>"
  Mux3/1 -> Bus Creator2/4  "MtrElecPwr"
  Memory/1 -> Bus Creator1/1  "Curr"
  MtrSpd/1 -> Mux1/1, Mapped Motor/2
  connections:
  Batt/RConn1 -- Two-Way Connection1/RConn1

== system EvBoltCalib_Lat_v1_comb/Vehicle/Powertrain Supervisory Controller  ==
  Driver : Inport
  Chassis : Inport  Port=2
  Mtr : Inport  Port=3
  Batt : Inport  Port=4
  Bus Selector : BusSelector  OutputSignals=SteeringCmd
  Engine Torque Command : Subsystem
  Subsystem1 : Subsystem
      mask Display: disp('')
  Subsystem4 : Subsystem
      mask Display: disp('')
  SupvsryCtrl : Outport
  wires:
  Engine Torque Command/4(DriverGearCmd) -> Subsystem1/4(DriverGearCmd)
  Engine Torque Command/3(BrkCmd) -> Subsystem1/3(BrkCmd)
  Engine Torque Command/2(AccelCmd) -> Subsystem1/2(AccelCmd)
  Engine Torque Command/1(MtrTrqCmd) -> Subsystem1/1(MtrTrqCmd)
  Subsystem4/6(MtrSpd) -> Engine Torque Command/6(MtrSpd)
  Subsystem4/5(BattSoc) -> Engine Torque Command/5(BattSoc)
  Subsystem4/4(VehSpd) -> Engine Torque Command/4(VehSpd)
  Subsystem4/3(DriverGearCmd) -> Engine Torque Command/3(DriverGearCmdIn)
  Mtr/1 -> Subsystem4/4(Mtr)
  Subsystem1/1(SupvsryCtrl) -> SupvsryCtrl/1
  Batt/1 -> Subsystem4/3(Batt)
  Chassis/1 -> Subsystem4/2(Chassis)
  Driver/1 -> Bus Selector/1, Subsystem4/1(Driver)
  Subsystem4/1(AccelCmd) -> Engine Torque Command/1(AccelCmdIn)
  Subsystem4/2(DecelCmd) -> Engine Torque Command/2(DecelCmdIn)
  Bus Selector/1 -> Subsystem1/5(SteeringCmd)  "<SteeringCmd>"

== system EvBoltCalib_Lat_v1_comb/Vehicle/Vehicle Dynamics ==
  Env : Inport
  SupvsryCtrl : Inport  Port=2
  AxlTrq : Inport  Port=3
  Vehicle 14DOF : Subsystem  VariantControl=Veh14DOF
  Vehicle 7DOF : Subsystem  VariantControl=Veh7DOF
  Vehicle Longitudinal : Subsystem  VariantControl=VehLong
  Whl : Outport
  Chassis : Outport  Port=2

== system EvBoltCalib_Lat_v1_comb/Driver/Direct Command From Reference/Subsystem1 ==
  AccelCmd : Inport
  DecelCmd : Inport  Port=2
  GearCmd : Inport  Port=3
  CltchCmd : Inport  Port=4
  IgSw : Inport  Port=5
  SteeringCmd : Inport  Port=6
  Bus Creator : BusCreator  Inputs=6
  TransPlant : Outport
  wires:
  AccelCmd/1 -> Bus Creator/1  "AccelCmd"
  DecelCmd/1 -> Bus Creator/2  "DecelCmd"
  Bus Creator/1 -> TransPlant/1  "Driver"
  GearCmd/1 -> Bus Creator/3  "GearCmd"
  CltchCmd/1 -> Bus Creator/4  "CltchCmd"
  IgSw/1 -> Bus Creator/5  "IgSw"
  SteeringCmd/1 -> Bus Creator/6  "SteeringCmd"

== system EvBoltCalib_Lat_v1_comb/Driver/Direct Command From Reference/Subsystem2 ==
  Env : Inport
  Veh : Inport  Port=2
  Terminator1 : Terminator
  Terminator2 : Terminator
  wires:
  Env/1 -> Terminator1/1
  Veh/1 -> Terminator2/1

== system EvBoltCalib_Lat_v1_comb/Driver/Open Loop Driver/Longitudinal Driver ==
  AccelCmdIn : Inport
  DecelCmdIn : Inport  Port=2
  Constant : Constant
  Constant1 : Constant
  Constant2 : Constant  Value=0
  AccelCmd : Outport
  DecelCmd : Outport  Port=2
  GearCmd : Outport  Port=3
  CltchCmd : Outport  Port=4
  IgSw : Outport  Port=5
  wires:
  Constant1/1 -> GearCmd/1
  Constant/1 -> IgSw/1
  DecelCmdIn/1 -> DecelCmd/1
  Constant2/1 -> CltchCmd/1
  AccelCmdIn/1 -> AccelCmd/1

== system EvBoltCalib_Lat_v1_comb/Driver/Open Loop Driver/Subsystem1 ==
  AccelCmd : Inport
  DecelCmd : Inport  Port=2
  GearCmd : Inport  Port=3
  CltchCmd : Inport  Port=4
  IgSw : Inport  Port=5
  SteeringCmd : Inport  Port=6
  Bus Creator : BusCreator  Inputs=6
  TransPlant : Outport
  wires:
  AccelCmd/1 -> Bus Creator/1  "AccelCmd"
  DecelCmd/1 -> Bus Creator/2  "DecelCmd"
  Bus Creator/1 -> TransPlant/1  "Driver"
  GearCmd/1 -> Bus Creator/3  "GearCmd"
  CltchCmd/1 -> Bus Creator/4  "CltchCmd"
  IgSw/1 -> Bus Creator/5  "IgSw"
  SteeringCmd/1 -> Bus Creator/6  "SteeringCmd"

== system EvBoltCalib_Lat_v1_comb/Driver/Open Loop Driver/Subsystem2 ==
  TestScnrio : Inport
  Env : Inport  Port=2
  Veh : Inport  Port=3
  Bus Selector : BusSelector  OutputSignals=AccelCmd,DecelCmd
  Terminator : Terminator
  Terminator1 : Terminator
  AccelCmd : Outport
  DecelCmd : Outport  Port=2
  wires:
  Bus Selector/1 -> AccelCmd/1  "<AccelCmd>"
  TestScnrio/1 -> Bus Selector/1
  Bus Selector/2 -> DecelCmd/1  "<DecelCmd>"
  Env/1 -> Terminator/1
  Veh/1 -> Terminator1/1

== system EvBoltCalib_Lat_v1_comb/Driver/Predictive Longitudinal Driver/Longitudinal Driver ==
  VehRefSpd : Inport
  VehRefSpdLookAhead : Inport  Port=2
  VehDistLookAhead : Inport  Port=3
  TimeLookAhead : Inport  Port=4
  VehSpd : Inport  Port=5
  VehDist : Inport  Port=6
  RoadGrade : Inport  Port=7
  GradeLookAhead : Inport  Port=8
  Constant : Constant
  Constant1 : Constant
  Constant2 : Constant  Value=0
  Longitudinal Predictive Driver : VsrLibDriver/Longitudinal Predictive Driver  VehMass=ChassisVehMass  aR=DriverLongLossA  bR=DriverLongLossB  cR=DriverLongLossC  MaxAccelFrcSpdBpts=DriverMaxAccelFrcSpdBpts  MaxAccelFrcTbl=DriverMaxAccelFrcTbl  AccelPdlBpts=DriverAccelPdlBpts  AccelPdlTbl=DriverAccelPdlTbl  BrakePdlBpts=DriverBrakePdlBpts  BrakeFrcTbl=DriverBrakeFrcTbl  SmoothTimeAvg=DriverSmoothTimeAvg  VelThresh=DriverVelThresh  PdlRateLimitWeight=DriverPdlRateLimitWeight  DistOptWeight=DriverDistOptWeight  NumOptimIters=DriverNumOptimIters  g=EnvGravCnst
  Terminator3 : Terminator
  Terminator4 : Terminator
  AccelCmd : Outport
  DecelCmd : Outport  Port=2
  GearCmd : Outport  Port=3
  CltchCmd : Outport  Port=4
  IgSw : Outport  Port=5
  wires:
  VehRefSpd/1 -> Terminator4/1
  RoadGrade/1 -> Terminator3/1
  VehSpd/1 -> Longitudinal Predictive Driver/4
  Constant/1 -> IgSw/1
  Constant1/1 -> GearCmd/1
  GradeLookAhead/1 -> Longitudinal Predictive Driver/6
  VehRefSpdLookAhead/1 -> Longitudinal Predictive Driver/1
  TimeLookAhead/1 -> Longitudinal Predictive Driver/3
  Longitudinal Predictive Driver/1 -> AccelCmd/1
  Longitudinal Predictive Driver/2 -> DecelCmd/1
  Constant2/1 -> CltchCmd/1
  VehDistLookAhead/1 -> Longitudinal Predictive Driver/2
  VehDist/1 -> Longitudinal Predictive Driver/5

== system EvBoltCalib_Lat_v1_comb/Driver/Predictive Longitudinal Driver/Subsystem1 ==
  AccelCmd : Inport
  DecelCmd : Inport  Port=2
  GearCmd : Inport  Port=3
  CltchCmd : Inport  Port=4
  IgSw : Inport  Port=5
  SteeringCmd : Inport  Port=6
  Bus Creator : BusCreator  Inputs=6
  TransPlant : Outport
  wires:
  AccelCmd/1 -> Bus Creator/1  "AccelCmd"
  DecelCmd/1 -> Bus Creator/2  "DecelCmd"
  Bus Creator/1 -> TransPlant/1  "Driver"
  GearCmd/1 -> Bus Creator/3  "GearCmd"
  CltchCmd/1 -> Bus Creator/4  "CltchCmd"
  IgSw/1 -> Bus Creator/5  "IgSw"
  SteeringCmd/1 -> Bus Creator/6  "SteeringCmd"

== system EvBoltCalib_Lat_v1_comb/Driver/Predictive Longitudinal Driver/Subsystem2 ==
  TestScnrio : Inport
  Env : Inport  Port=2
  Veh : Inport  Port=3
  Bus Selector : BusSelector  OutputSignals=VehRefSpd,VehRefSpdLookAhead,VehDistLookAhead,VehDist,GradeLookAhead,TimeLookAhead
  Bus Selector1 : BusSelector  OutputSignals=RoadGrade
  Bus Selector2 : BusSelector  OutputSignals=Chassis.VehSpd
  VehRefSpd : Outport
  VehRefSpdLookAhead : Outport  Port=2
  VehDistLookAhead : Outport  Port=3
  TimeLookAhead : Outport  Port=4
  VehSpd : Outport  Port=5
  VehDist : Outport  Port=6
  RoadGrade : Outport  Port=7
  GradeLookAhead : Outport  Port=8
  wires:
  TestScnrio/1 -> Bus Selector/1
  Env/1 -> Bus Selector1/1
  Bus Selector1/1 -> RoadGrade/1  "<RoadGrade>"
  Veh/1 -> Bus Selector2/1
  Bus Selector2/1 -> VehSpd/1  "<VehSpd>"
  Bus Selector/1 -> VehRefSpd/1  "<VehRefSpd>"
  Bus Selector/2 -> VehRefSpdLookAhead/1  "<VehRefSpdLookAhead>"
  Bus Selector/3 -> VehDistLookAhead/1  "<VehDistLookAhead>"
  Bus Selector/4 -> VehDist/1  "<VehDist>"
  Bus Selector/5 -> GradeLookAhead/1  "<GradeLookAhead>"
  Bus Selector/6 -> TimeLookAhead/1  "<TimeLookAhead>"
